simulink model "CCModel_73"  (R2024a)
settings: Solver=ode3  StartTime=0.0  StopTime=100  FixedStep=0.001  RelTol=1e-3  EnableMultiTasking=on
undefined symbols (not defined in the file or in its folder): DiscIntNeverNeededParam, Hecate_desVel1, Hecate_desVel2, Hecate_desVel3, Hecate_horShift, Hecate_period, Hecate_slope, Hecate_Transition1, Hecate_Transition2, Hecate_verShift, i, PME_qb, qb_map, RPM_qb, V
libraries: simulink x46
(part 2 of 11)

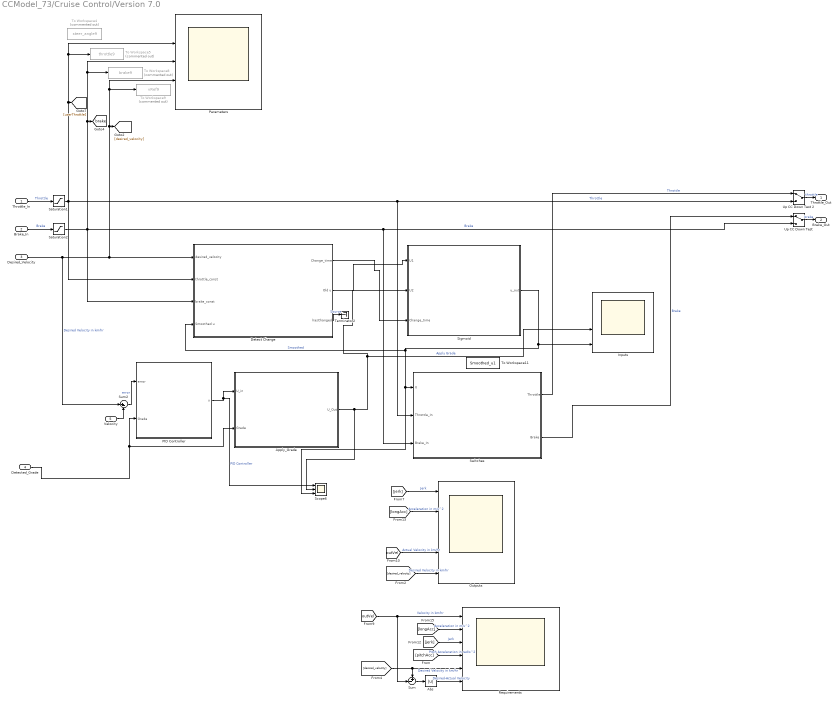
== system CCModel_73/Cruise Control/Version 7.0 ==
  Throttle_In : Inport
  Brake_In : Inport  Port=2
  Desired_Velocity : Inport  Port=3
  Detected_Grade : Inport  Port=4
  Velocity : Inport  Port=5
  Abs : Abs  SaturateOnIntegerOverflow=off
  Apply_Grade : Subsystem
  Detect Change : Subsystem
  Inputs : Scope  NumInputPorts=4
  Outputs : Scope  NumInputPorts=5
  PID Controller : Subsystem
  Parameters : Scope  NumInputPorts=5
  Requirements : Scope  NumInputPorts=6
  Saturation1 : Saturate  UpperLimit=100  LowerLimit=-100
  Saturation2 : Saturate  UpperLimit=100  LowerLimit=-100
  Scope6 : Scope  NumInputPorts=3
  Sigmoid : Subsystem
  Sum : Sum  Inputs=+-|
  Sum2 : Sum  Inputs=|+-
  Switches : Subsystem
  Terminator2 : Terminator
  To Workspace11 : ToWorkspace  VariableName=Smoothed_u1  SampleTime=-1
  To Workspace4 : ToWorkspace  Commented=on  VariableName=steer_angle9  SampleTime=-1
      settings: Save2DSignal=2-D array (concatenate along first dimension)
  To Workspace5 : ToWorkspace  Commented=on  VariableName=throttle9  SampleTime=-1
      settings: Save2DSignal=2-D array (concatenate along first dimension)
  To Workspace8 : ToWorkspace  Commented=on  VariableName=brake9  SampleTime=-1
      settings: Save2DSignal=2-D array (concatenate along first dimension)
  To Workspace9 : ToWorkspace  Commented=on  VariableName=vRef9  SampleTime=-1
      settings: Save2DSignal=2-D array (concatenate along first dimension)
  Up CC Down Test : ManualSwitch
  Up CC Down Test 2 : ManualSwitch
  Throttle_Out : Outport
  Brake_Out : Outport  Port=2
  tag scope: brake=global
  wires:
  Abs/1 -> Requirements/6  "Desired-Actual Velocity"
  Sum/1 -> Abs/1
  Switches/2(Brake) -> Up CC Down Test/1  "Brake"
  Saturation2/1 -> Switches/3(Brake_In), Up CC Down Test/2, Detect Change/3(brake_const), To Workspace8/1, Parameters/3, [brake]  "Brake"
  [jerk] -> Requirements/3  "Jerk"
  Detect Change/1(Change_time) -> Sigmoid/3(Change_time)
  Desired_Velocity/1 -> To Workspace9/1, Parameters/4, [desired_velocity], Detect Change/1(desired_velocity), Sum2/1  "Desired Velocity in km/hr"
  Sum2/1 -> PID Controller/1(error)  "error"
  Switches/1(Throttle) -> Up CC Down Test 2/1  "Throttle"
  PID Controller/1(u) -> Scope6/1, Apply_Grade/1(U_in)  "PID Controller"
  [outVel] -> Outputs/4  "Actual Velocity in km/hr"
  [longAcc] -> Outputs/2  "Acceleration in m/s^2"
  Throttle_In/1 -> Saturation1/1  "Throttle"
  [desired_velocity] -> Outputs/5  "Desired Velocity in km/hr"
  [longAcc] -> Requirements/2  "Acceleration in m/s^2"
  Up CC Down Test 2/1 -> Throttle_Out/1  "throttle"
  Velocity/1 -> Sum2/2
  [desired_velocity] -> Sum/1, Requirements/5  "Desired Velocity in km/hr"
  Detected_Grade/1 -> Apply_Grade/2(Grade), PID Controller/2(Grade)
  Brake_In/1 -> Saturation2/1  "Brake"
  Detect Change/3(hasChanged) -> Terminator2/1  "Source"
  Detect Change/2(Old u) -> Sigmoid/1(U1)
  Sigmoid/1(u_out) -> Detect Change/4(Smoothed u), Scope6/3, Switches/1(U), Inputs/4  "Smoothed"
  Apply_Grade/1(U_Out) -> Scope6/2, Inputs/3, Sigmoid/2(U2)  "Apply Grade"
  [pitchAcc] -> Requirements/4  "Pitch Acceleration in rad/s^2"
  [jerk] -> Outputs/1  "Jerk"
  Saturation1/1 -> Switches/2(Throttle_In), Up CC Down Test 2/2, Detect Change/2(throttle_const), [userThrottle], Parameters/2, To Workspace5/1  "Throttle"
  [outVel] -> Sum/2, Requirements/1  "Velocity in km/hr"
  Up CC Down Test/1 -> Brake_Out/1  "brake"

== system CCModel_73/Cruise Control/Version 7.1 ==
  Throttle_In : Inport
  Brake_In : Inport  Port=2
  Desired_Velocity : Inport  Port=3
  Detected_Grade : Inport  Port=4
  Velocity : Inport  Port=5
  Abs : Abs  SaturateOnIntegerOverflow=off
  Apply_Grade : Subsystem
  Detect Change : Subsystem
  Inputs : Scope  NumInputPorts=4
  Outputs : Scope  NumInputPorts=5
  PID Controller : Subsystem
  Parameters : Scope  NumInputPorts=5
  Requirements : Scope  NumInputPorts=6
  Saturation1 : Saturate  UpperLimit=100  LowerLimit=-100
  Saturation2 : Saturate  UpperLimit=100  LowerLimit=-100
  Scope6 : Scope  NumInputPorts=3
  Sigmoid : Subsystem
  Sum : Sum  Inputs=+-|
  Sum2 : Sum  Inputs=|+-
  Switches : Subsystem
  To Workspace4 : ToWorkspace  Commented=on  VariableName=steer_angle10  SampleTime=-1
      settings: Save2DSignal=2-D array (concatenate along first dimension)
  To Workspace5 : ToWorkspace  Commented=on  VariableName=throttle10  SampleTime=-1
      settings: Save2DSignal=2-D array (concatenate along first dimension)
  To Workspace8 : ToWorkspace  Commented=on  VariableName=brake10  SampleTime=-1
      settings: Save2DSignal=2-D array (concatenate along first dimension)
  To Workspace9 : ToWorkspace  Commented=on  VariableName=vRef10  SampleTime=-1
      settings: Save2DSignal=2-D array (concatenate along first dimension)
  Up CC Down Test : ManualSwitch
  Up CC Down Test 2 : ManualSwitch
  Throttle_Out : Outport
  Brake_Out : Outport  Port=2
  tag scope: ChangeTrigger=global, brake=global
  wires:
  PID Controller/1(u) -> Scope6/1, Apply_Grade/1(U_in)  "PID Controller"
  Detect Change/2(Old u) -> Sigmoid/1(U1)
  [longAcc] -> Outputs/2  "Acceleration in m/s^2"
  [desired_velocity] -> Outputs/5  "Desired Velocity in km/hr"
  Up CC Down Test 2/1 -> Throttle_Out/1  "throttle"
  Detect Change/1(Change_time) -> Sigmoid/3(Change_time)
  [outVel] -> Outputs/4  "Actual Velocity in km/hr"
  [desired_velocity] -> Sum/1, Requirements/5  "Desired Velocity in km/hr"
  [outVel] -> Sum/2, Requirements/1  "Velocity in km/hr"
  Velocity/1 -> Sum2/2
  [longAcc] -> Requirements/2  "Acceleration in m/s^2"
  Throttle_In/1 -> Saturation1/1  "Throttle"
  Abs/1 -> Requirements/6  "Desired-Actual Velocity"
  Switches/2(Brake) -> Up CC Down Test/1  "Brake"
  Sum/1 -> Abs/1
  Saturation2/1 -> Switches/3(Brake_In), Up CC Down Test/2, Detect Change/3(brake_const), To Workspace8/1, Parameters/3, [brake]  "Brake"
  Apply_Grade/1(U_Out) -> Scope6/2, Inputs/3, Sigmoid/2(U2)  "Apply Grade"
  [jerk] -> Requirements/3  "Jerk"
  [jerk] -> Outputs/1  "Jerk"
  Detect Change/3(hasChanged) -> [ChangeTrigger]  "Source"
  [pitchAcc] -> Requirements/4  "Pitch Acceleration in rad/s^2"
  Sum2/1 -> PID Controller/1(error)  "error"
  Switches/1(Throttle) -> Up CC Down Test 2/1  "Throttle"
  Brake_In/1 -> Saturation2/1  "Brake"
  Sigmoid/1(u_out) -> Detect Change/4(Smoothed u), Scope6/3, Switches/1(U), Inputs/4  "Smoothed"
  Desired_Velocity/1 -> To Workspace9/1, Parameters/4, [desired_velocity], Detect Change/1(desired_velocity), Sum2/1  "Desired Velocity in km/hr"
  Saturation1/1 -> [userThrottle], Parameters/2, To Workspace5/1, Switches/2(Throttle_In), Up CC Down Test 2/2, Detect Change/2(throttle_const)  "Throttle"
  Detected_Grade/1 -> Apply_Grade/2(Grade), PID Controller/2(Grade)
  Up CC Down Test/1 -> Brake_Out/1  "brake"

== system CCModel_73/Cruise Control/Version 7.2 ==
  Throttle_In : Inport
  Brake_In : Inport  Port=2
  Desired_Velocity : Inport  Port=3
  Detected_Grade : Inport  Port=4
  Velocity : Inport  Port=5
  Abs : Abs  SaturateOnIntegerOverflow=off
  Apply_Grade : Subsystem
  Detect Change : Subsystem
  Inputs : Scope  NumInputPorts=4
  PID Controller : Subsystem
  Parameters : Scope  NumInputPorts=5
  Requirements : Scope  NumInputPorts=6
  Saturation1 : Saturate  UpperLimit=100  LowerLimit=-100
  Saturation2 : Saturate  UpperLimit=100  LowerLimit=-100
  Scope6 : Scope  NumInputPorts=3
  Scope7 : Scope  NumInputPorts=5
  Sigmoid : Subsystem
  Sum : Sum  Inputs=+-|
  Sum2 : Sum  Inputs=|+-
  Switches : Subsystem
  To Workspace4 : ToWorkspace  Commented=on  VariableName=steer_angle11  SampleTime=-1
      settings: Save2DSignal=2-D array (concatenate along first dimension)
  To Workspace5 : ToWorkspace  Commented=on  VariableName=throttle11  SampleTime=-1
      settings: Save2DSignal=2-D array (concatenate along first dimension)
  To Workspace8 : ToWorkspace  Commented=on  VariableName=brake11  SampleTime=-1
      settings: Save2DSignal=2-D array (concatenate along first dimension)
  To Workspace9 : ToWorkspace  Commented=on  VariableName=vRef11  SampleTime=-1
      settings: Save2DSignal=2-D array (concatenate along first dimension)
  Up CC Down Test : ManualSwitch
  Up CC Down Test 2 : ManualSwitch
  Throttle_Out : Outport
  Brake_Out : Outport  Port=2
  tag scope: brake=global
  wires:
  [jerk] -> Scope7/1  "Jerk"
  [outVel] -> Scope7/4  "Actual Velocity in km/hr"
  [pitchAcc] -> Requirements/4  "Pitch Acceleration in rad/s^2"
  Up CC Down Test 2/1 -> Throttle_Out/1  "throttle"
  [longAcc] -> Requirements/2  "Acceleration in m/s^2"
  [outVel] -> Sum/2, Requirements/1  "Velocity in km/hr"
  Saturation1/1 -> Switches/2(Throttle_In), Up CC Down Test 2/2, Detect Change/2(throttle_const), [userThrottle], Parameters/2, To Workspace5/1  "Throttle"
  Velocity/1 -> Sum2/2
  [desired_velocity] -> Sum/1, Requirements/5  "Desired Velocity in km/hr"
  Detect Change/1(Change_time) -> Sigmoid/3(Change_time)
  Switches/2(Brake) -> Up CC Down Test/1  "Brake"
  Sum2/1 -> PID Controller/1(error)  "error"
  Desired_Velocity/1 -> To Workspace9/1, Parameters/4, [desired_velocity], Detect Change/1(desired_velocity), Sum2/1  "Desired Velocity in km/hr"
  Throttle_In/1 -> Saturation1/1  "Throttle"
  Switches/1(Throttle) -> Up CC Down Test 2/1  "Throttle"
  Saturation2/1 -> Switches/3(Brake_In), Up CC Down Test/2, Detect Change/3(brake_const), To Workspace8/1, Parameters/3, [brake]  "Brake"
  Detected_Grade/1 -> Apply_Grade/2(Grade), PID Controller/2(Grade)
  Sigmoid/1(u_out) -> Detect Change/4(Smoothed u), Scope6/3, Switches/1(U), Inputs/4  "Smoothed"
  Abs/1 -> Requirements/6  "Desired-Actual Velocity"
  [longAcc] -> Scope7/2  "Acceleration in m/s^2"
  Detect Change/3(hasChanged) -> Sigmoid/4(hasChanged)  "Source"
  Sum/1 -> Abs/1
  Brake_In/1 -> Saturation2/1  "Brake"
  PID Controller/1(u) -> Scope6/1, Apply_Grade/1(U_in)  "PID Controller"
  Detect Change/2(Old u) -> Sigmoid/1(U1)
  [desired_velocity] -> Scope7/5  "Desired Velocity in km/hr"
  Apply_Grade/1(U_Out) -> Scope6/2, Inputs/3, Sigmoid/2(U2)  "Apply Grade"
  [jerk] -> Requirements/3  "Jerk"
  Up CC Down Test/1 -> Brake_Out/1  "brake"

== system CCModel_73/Cruise Control/Version 7.3 ==
  Throttle_In : Inport
  Brake_In : Inport  Port=2
  Desired_Velocity : Inport  Port=3
  Detected_Grade : Inport  Port=4
  Velocity : Inport  Port=5
  Abs : Abs  SaturateOnIntegerOverflow=off
  Apply_Grade : Subsystem
  Detect Change : Subsystem
  Inputs : Scope  NumInputPorts=4
  Outputs : Scope  NumInputPorts=5
  PID Controller : Subsystem
  Parameters : Scope  NumInputPorts=5
  Requirements : Scope  NumInputPorts=6
  Saturation1 : Saturate  UpperLimit=100  LowerLimit=-100
  Saturation2 : Saturate  UpperLimit=100  LowerLimit=-100
  Scope6 : Scope  NumInputPorts=3
  Sigmoid : Subsystem
  Sum : Sum  Inputs=+-|
  Sum2 : Sum  Inputs=|+-
  Switches : Subsystem
  To Workspace18 : ToWorkspace  VariableName=Jerk  SampleTime=-1
      settings: Save2DSignal=2-D array (concatenate along first dimension)
  To Workspace4 : ToWorkspace  Commented=on  VariableName=steer_angle12  SampleTime=-1
      settings: Save2DSignal=2-D array (concatenate along first dimension)
  To Workspace5 : ToWorkspace  Commented=on  VariableName=throttle13  SampleTime=-1
      settings: Save2DSignal=2-D array (concatenate along first dimension)
  To Workspace8 : ToWorkspace  Commented=on  VariableName=brake12  SampleTime=-1
      settings: Save2DSignal=2-D array (concatenate along first dimension)
  To Workspace9 : ToWorkspace  Commented=on  VariableName=vRef12  SampleTime=-1
      settings: Save2DSignal=2-D array (concatenate along first dimension)
  Up CC Down Test : ManualSwitch
  Up CC Down Test 2 : ManualSwitch
  Throttle_Out : Outport
  Brake_Out : Outport  Port=2
  tag scope: ChangeTrigger=global, brake=global
  wires:
  Velocity/1 -> Sum2/2
  Sum2/1 -> Detect Change/5(error), PID Controller/1(Error)  "error"
  [jerk] -> Outputs/1  "Jerk"
  Switches/2(Brake) -> Up CC Down Test/1  "Brake"
  Switches/1(Throttle) -> Up CC Down Test 2/1  "Throttle"
  PID Controller/1(u) -> Scope6/1, Apply_Grade/1(U_in)  "PID Controller"
  Detect Change/3(hasChanged) -> PID Controller/2(Source)  "Source"
  [outVel] -> Outputs/4  "Actual Velocity in km/hr"
  [longAcc] -> Outputs/2  "Acceleration in m/s^2"
  [longAcc] -> Requirements/2  "Acceleration in m/s^2"
  Abs/1 -> Requirements/6  "Desired-Actual Velocity"
  [pitchAcc] -> Requirements/4  "Pitch Acceleration in rad/s^2"
  [jerk] -> To Workspace18/1, Requirements/3  "Jerk"
  [desired_velocity] -> Sum/1, Requirements/5  "Desired Velocity in km/hr"
  Saturation2/1 -> Switches/3(Brake_In), Up CC Down Test/2, Detect Change/3(brake_const), To Workspace8/1, Parameters/3, [brake]  "Brake"
  Detect Change/1(Change_time) -> Sigmoid/3(Change_time)
  [desired_velocity] -> Outputs/5  "Desired Velocity in km/hr"
  Detected_Grade/1 -> Apply_Grade/2(Grade)
  [outVel] -> Sum/2, Requirements/1  "Velocity in km/hr"
  Detect Change/2(Old u) -> Sigmoid/1(U1)  "Original"
  Brake_In/1 -> Saturation2/1  "Brake"
  Throttle_In/1 -> Saturation1/1  "Throttle"
  Sum/1 -> Abs/1
  Desired_Velocity/1 -> To Workspace9/1, Parameters/4, [desired_velocity], Detect Change/1(desired_velocity), PID Controller/3(Desired Velocity), Sum2/1  "Desired Velocity in km/hr"
  Up CC Down Test 2/1 -> Throttle_Out/1  "throttle"
  Sigmoid/1(u_out) -> Detect Change/4(Smoothed u), Scope6/3, Switches/1(U), Inputs/4  "Smoothed"
  Saturation1/1 -> Switches/2(Throttle_In), Up CC Down Test 2/2, Detect Change/2(throttle_const), [userThrottle], Parameters/2, To Workspace5/1  "Throttle"
  Apply_Grade/1(U_Out) -> Scope6/2, Inputs/3, Sigmoid/2(U2)  "Original"
  Up CC Down Test/1 -> Brake_Out/1  "brake"
  Detect Change/4(ChangeTrigger) -> [ChangeTrigger]

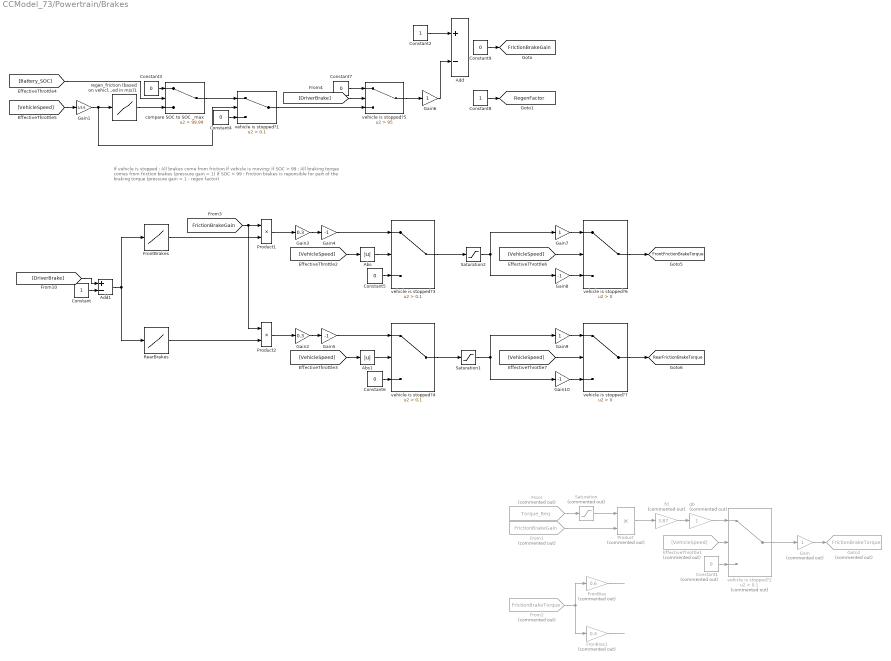
== system CCModel_73/Powertrain/Brakes ==
  note: If vehicle is stopped : All brakes come from friction
      | If vehicle is moving:
      | If SOC > 99 : All braking torque comes from friction brakes (pressure gain = 1)
      | If SOC < 99 : Friction brakes is reponsible for part of the braking torque (pressure gain = 1 - regen factor)
  Abs : Abs  SaturateOnIntegerOverflow=off
  Abs1 : Abs  SaturateOnIntegerOverflow=off
  Add : Sum  Inputs=+-
  Add1 : Sum  Inputs=+-
  Constant : Constant
  Constant1 : Constant  Commented=on  Value=0
  Constant2 : Constant
  Constant{3..7,9} (6 alike) : Constant  Value=0
  Constant8 : Constant
  EffectiveThrottle1 : From  Commented=on  GotoTag=VehicleSpeed  TagVisibility=global
      settings: CloseFcn=tagdialog Close
  From : From  Commented=on  GotoTag=Torque_Req  TagVisibility=global
  From1 : From  Commented=on  GotoTag=FrictionBrakeGain  TagVisibility=global
  From2 : From  Commented=on  GotoTag=FrictionBrakeTorque  TagVisibility=global
  FronBias : Gain  Commented=on  Gain=0.6
  FronBias1 : Gain  Commented=on  Gain=0.4
  FrontBrakes : Lookup_n-D  NumberOfTableDimensions=1  BreakpointsForDimension1=[0 10 20 30 40 50 60 70 80 90 100]  Table=[0 520 960 1390 1830 2260 2700 3140 3590 4030 4475]  InternalRulePriority=Speed  RndMeth=Simplest
  Gain : Gain  Commented=on
  Gain1 : Gain  Gain=1/3.6
  Gain{4..5,8,10} (4 alike) : Gain  Gain=-1
  Gain2 : Gain  Gain=0.3
  Gain3 : Gain  Gain=0.3
  Gain6 : Gain
  Gain7 : Gain
  Gain9 : Gain
  Goto2 : Goto  Commented=on  GotoTag=FrictionBrakeTorque  TagVisibility=global
  Product : Product  Commented=on
  Product1 : Product
  Product2 : Product
  RearBrakes : Lookup_n-D  NumberOfTableDimensions=1  BreakpointsForDimension1=[0 10 20 30 40 50 60 70 80 90 100]  Table=[0 170 250 340 420 500 580 664 740 825 905]  InternalRulePriority=Speed  RndMeth=Simplest
  Saturation : Saturate  Commented=on  UpperLimit=0  LowerLimit=-inf
  Saturation1 : Saturate  UpperLimit=0  LowerLimit=-inf
  Saturation2 : Saturate  UpperLimit=0  LowerLimit=-inf
  compare SOC to SOC _max : Switch  Criteria=u2 > Threshold  Threshold=99.99  SaturateOnIntegerOverflow=off  InputSameDT=off
  fd : Gain  Commented=on  Gain=3.87
  gb : Gain  Commented=on
  regen_friction (based on vehicle speed in m/s)1 : Lookup_n-D  NumberOfTableDimensions=1  BreakpointsForDimension1=[0,2.76,5.55,8.31,11.07,13.83,16.68,27.76,300]  Table="[0\t0.25  0.25\t0.25\t  0.50\t0.95\t0.95\t0.95   0.95]"  InternalRulePriority=Speed  RndMeth=Simplest
  vehicle is stopped?1 : Switch  Criteria=u2 > Threshold  Threshold=0.1  SaturateOnIntegerOverflow=off  InputSameDT=off
  vehicle is stopped?2 : Switch  Commented=on  Criteria=u2 > Threshold  Threshold=0.1  SaturateOnIntegerOverflow=off  InputSameDT=off
  vehicle is stopped?3 : Switch  Criteria=u2 > Threshold  Threshold=0.1  SaturateOnIntegerOverflow=off  InputSameDT=off
  vehicle is stopped?4 : Switch  Criteria=u2 > Threshold  Threshold=0.1  SaturateOnIntegerOverflow=off  InputSameDT=off
  vehicle is stopped?5 : Switch  Criteria=u2 > Threshold  Threshold=95  SaturateOnIntegerOverflow=off  InputSameDT=off
  vehicle is stopped?6 : Switch  Criteria=u2 > Threshold  SaturateOnIntegerOverflow=off  InputSameDT=off
  vehicle is stopped?7 : Switch  Criteria=u2 > Threshold  SaturateOnIntegerOverflow=off  InputSameDT=off
  tag scope: FrictionBrakeGain=global, FrontFrictionBrakeTorque=global, RearFrictionBrakeTorque=global, RegenFactor=global
  wires:
  [VehicleSpeed] -> Gain1/1
  Gain1/1 -> vehicle is stopped?1/2, regen_friction (based on vehicle speed in m/s)1/1
  Constant2/1 -> Add/1
  Constant3/1 -> compare SOC to SOC _max/1
  compare SOC to SOC _max/1 -> vehicle is stopped?1/1
  [Battery_SOC] -> compare SOC to SOC _max/2
  Constant4/1 -> vehicle is stopped?1/3
  EffectiveThrottle1/1 -> vehicle is stopped?2/2
  From1/1 -> Product/2
  fd/1 -> gb/1
  FronBias/1 -> ?
  FronBias1/1 -> ?
  From2/1 -> FronBias/1, FronBias1/1
  Saturation/1 -> Product/1
  gb/1 -> vehicle is stopped?2/1
  Constant1/1 -> vehicle is stopped?2/3
  vehicle is stopped?2/1 -> Gain/1
  From/1 -> Saturation/1
  Product/1 -> fd/1
  Gain/1 -> Goto2/1
  regen_friction (based on vehicle speed in m/s)1/1 -> compare SOC to SOC _max/3
  Add1/1 -> RearBrakes/1, FrontBrakes/1
  FrontBrakes/1 -> Product1/2
  RearBrakes/1 -> Product2/2
  [FrictionBrakeGain] -> Product2/1, Product1/1
  Product1/1 -> Gain3/1
  Product2/1 -> Gain2/1
  Gain2/1 -> Gain5/1
  Gain3/1 -> Gain4/1
  Constant/1 -> Add1/2
  [DriverBrake] -> Add1/1
  Gain6/1 -> Add/2
  [DriverBrake] -> vehicle is stopped?5/2
  vehicle is stopped?1/1 -> vehicle is stopped?5/3
  Constant7/1 -> vehicle is stopped?5/1
  vehicle is stopped?5/1 -> Gain6/1
  Abs1/1 -> vehicle is stopped?4/2
  Constant5/1 -> vehicle is stopped?3/3
  vehicle is stopped?7/1 -> [RearFrictionBrakeTorque]
  [VehicleSpeed] -> vehicle is stopped?7/2
  Gain10/1 -> vehicle is stopped?7/3
  Saturation1/1 -> Gain9/1, Gain10/1
  Saturation2/1 -> Gain8/1, Gain7/1
  Gain8/1 -> vehicle is stopped?6/3
  [VehicleSpeed] -> vehicle is stopped?6/2
  vehicle is stopped?4/1 -> Saturation1/1
  Gain9/1 -> vehicle is stopped?7/1
  Gain4/1 -> vehicle is stopped?3/1
  vehicle is stopped?3/1 -> Saturation2/1
  Gain7/1 -> vehicle is stopped?6/1
  Constant6/1 -> vehicle is stopped?4/3
  Abs/1 -> vehicle is stopped?3/2
  Gain5/1 -> vehicle is stopped?4/1
  vehicle is stopped?6/1 -> [FrontFrictionBrakeTorque]
  [VehicleSpeed] -> Abs/1
  [VehicleSpeed] -> Abs1/1
  Constant8/1 -> [RegenFactor]
  Constant9/1 -> [FrictionBrakeGain]

== system CCModel_73/Powertrain/Central Differential ==
  0 : Constant
  "1 " : Constant  Value=0
  Add : Sum  Inputs=+++
  Central Differential Active : Constant  Value=CentralDifferentialActive
  Constant : Constant
  Front Bias : Constant  Value=FrontBias
  Gain : Gain  Gain=0.5
  Gain1 : Gain  Gain=0.5
  Gain2 : Gain  Gain=0.5
  Product : Product
  Product1 : Product
  Sum : Sum  Inputs=-+|
  Sum1 : Sum
  Sum2 : Sum
  Sum3 : Sum
  Switch : Switch  Criteria=u2 > Threshold  SaturateOnIntegerOverflow=off  InputSameDT=off
  prod{,1..4} (5 alike) : Product
  tag scope: DiffFrontInputTorque=global, DiffRearInputTorque=global, GearboxOutputAlpha=global, GearboxOutputAngle=global, GearboxOutputOmega=global, InternalCentralDiffActivity=global
  wires:
  Front Bias/1 -> Sum/1, Product/2
  Constant/1 -> Sum/2
  Sum/1 -> Product1/2
  Add/1 -> Product1/1, Product/1
  Sum1/1 -> Gain/1
  [DiffRearInputOmega] -> Sum1/2
  [DiffFrontInputOmega] -> Sum1/1
  Sum2/1 -> Gain1/1
  [DiffRearInputAlpha] -> Sum2/2
  [DiffFrontInputAlpha] -> Sum2/1
  Sum3/1 -> Gain2/1
  [DiffRearInputAngle] -> Sum3/2
  [DiffFrontInputAngle] -> Sum3/1
  Central Differential Active/1 -> Switch/2, prod4/1, prod3/1, prod2/1, prod1/1, prod/1
  prod1/1 -> [DiffRearInputTorque]
  prod2/1 -> [GearboxOutputOmega]
  prod3/1 -> [GearboxOutputAlpha]
  prod4/1 -> [GearboxOutputAngle]
  Product/1 -> prod/2
  Product1/1 -> prod1/2
  Gain/1 -> prod2/2
  Gain1/1 -> prod3/2
  Gain2/1 -> prod4/2
  Switch/1 -> [InternalCentralDiffActivity]
  "1 "/1 -> Switch/1
  0/1 -> Switch/3
  [EM3Torque] -> Add/2
  [EVTorque] -> Add/3
  [DiffCenterInputshaftTorque] -> Add/1
  prod/1 -> [DiffFrontInputTorque]

== system CCModel_73/Powertrain/Clutch ==
  0 : Constant
  "1 " : Constant  Value=0
  Add : Sum  Inputs=+++
  Clutch Active : Constant  Value=ClutchActive
  Clutch Closed : Constant
  Clutch Omega : Product
  Constant1 : Constant  Value=0
  Gearbox Omega : Product
  GearboxAlpha : From  Commented=on  GotoTag=GearboxAlpha  TagVisibility=global
      settings: CloseFcn=tagdialog Close
  GearboxAngle : From  Commented=on  GotoTag=GearboxAngle  TagVisibility=global
      settings: CloseFcn=tagdialog Close
  Inertia to Accel : Gain  Gain=1/0.1
  Saturation : Saturate  UpperLimit=0  LowerLimit=-1000000
  Scope : Scope  Commented=on  NumInputPorts=2
  Sum : Sum
  Sum1 : Sum  Inputs=|++
  Sum2 : Sum  Inputs=+-  SaturateOnIntegerOverflow=on
  Switch : Switch  Criteria=u2 > Threshold  SaturateOnIntegerOverflow=off  InputSameDT=off
  Torque : Product
  "Vicrt Integration Time Step " : Gain  Gain=0.001
  prod : Product
  prod1 : Product
  tag scope: ClutchInputAlpha=global, ClutchInputAngle=global, ClutchInputOmega=global, GearboxInputTorque=global, InternalClutchActivity=global
  wires:
  [ClutchDemand] -> Sum2/2, Clutch Omega/1
  Inertia to Accel/1 -> "Vicrt Integration Time Step "/1
  Clutch Closed/1 -> Sum2/1
  Sum2/1 -> Gearbox Omega/1, Torque/2
  Gearbox Omega/1 -> Sum/1
  [GearboxOmega] -> Gearbox Omega/2
  [EngineOmega] -> Clutch Omega/2
  Clutch Omega/1 -> Sum/2
  Add/1 -> Torque/1, Inertia to Accel/1
  Sum/1 -> Sum1/1
  "Vicrt Integration Time Step "/1 -> Saturation/1
  Saturation/1 -> Sum1/2
  GearboxAlpha/1 -> Scope/1
  GearboxAngle/1 -> Scope/2
  Constant1/1 -> [ClutchInputAlpha], [ClutchInputAngle]
  prod/1 -> [GearboxInputTorque]
  prod1/1 -> [ClutchInputOmega]
  Sum1/1 -> prod1/2
  Torque/1 -> prod/2
  Clutch Active/1 -> prod1/1, prod/1, Switch/2
  "1 "/1 -> Switch/1
  0/1 -> Switch/3
  Switch/1 -> [InternalClutchActivity]
  [ClutchInputplateTorque] -> Add/1
  [EM1Torque] -> Add/2
  [EM0Torque] -> Add/3

== system CCModel_73/Powertrain/EM0 ==
  note: If Torque is positive: Motor does its best
      | If torque is negative: Case 01: SOC > 99: No Regen (Tmot = 0)
      | Case 02: SOC < 99: Regen
      | If Vehicle is stopped: No Regen Brakes
  0 : Constant
  "1 " : Constant  Value=0
  Constant1 : Constant  Value=0
  EM0 Active : Constant  Value=EM0Active
  EM0ConectionRatio : Constant  Value=EM0_Ratio
  Memory1 : Memory  InheritSampleTime=on
  Negative Motor Torque Table : Lookup_n-D  NumberOfTableDimensions=1  BreakpointsForDimension1=|  Table=|  InternalRulePriority=Speed  RndMeth=Simplest
      BreakpointsForDimension1=|
      | [1
      | 300
      | 700
      | 1000
      | 1300
      | 1600
      | 1900
      | 2200
      | 2500
      | 2800
      | 3100
      | 3400
      | 3700
      | 4000
      | 4300
      | 4600
      | 4900
      | 5200
      | 5500
      | 5800
      | 6100
      | 6400
      | 6700
      | 7000
      | 7400
      | 7800
      | 8200
      | 8600
      | 8810]
      Table=|
      | [-360
      | -360
      | -360
      | -360
      | -360
      | -357.728404316261
      | -357.682405078656
      | -356.960983702214
      | -356.300227986961
      | -355.518140949330
      | -355.472141711725
      | -351.285699987009
      | -343.284814075766
      | -334.455149023278
      | -326.397812480700
      | -307.963362459085
      | -289.161940741908
      | -276.934802218937
      | -265.691686602383
      | -254.400604378871
      | -242.676261199004
      | -229.462130210989
      | -218.075437684875
      | -207.776256300937
      | -192.222891861329
      | -178.005775209291
      | -168.578005975641
      | -157.192637101830
      | -152.195121951219]
  Positive Motor Torque Table : Lookup_n-D  NumberOfTableDimensions=1  BreakpointsForDimension1=|  Table=|  InternalRulePriority=Speed  RndMeth=Simplest
      BreakpointsForDimension1=|
      | [1
      | 300
      | 700
      | 1000
      | 1300
      | 1600
      | 1900
      | 2200
      | 2500
      | 2800
      | 3100
      | 3400
      | 3700
      | 4000
      | 4300
      | 4600
      | 4900
      | 5200
      | 5500
      | 5800
      | 6100
      | 6400
      | 6700
      | 7000
      | 7400
      | 7800
      | 8200
      | 8600
      | 8810]
      Table=|
      | [360
      | 360
      | 360
      | 360
      | 360
      | 357.728404316261
      | 357.682405078656
      | 356.960983702214
      | 356.300227986961
      | 355.518140949330
      | 355.472141711725
      | 351.285699987009
      | 343.284814075766
      | 334.455149023278
      | 326.397812480700
      | 307.963362459085
      | 289.161940741908
      | 276.934802218937
      | 265.691686602383
      | 254.400604378871
      | 242.676261199004
      | 229.462130210989
      | 218.075437684875
      | 207.776256300937
      | 192.222891861329
      | 178.005775209291
      | 168.578005975641
      | 157.192637101830
      | 152.195121951219]
  Product : Product
  Saturation Dynamic1 : simulink/Discontinuities/Saturation Dynamic  OutMin=[-360]  OutMax=[360]  OutDataTypeStr=Inherit: Same as second input  OutDataType=fixdt(1, 16)  OutScaling=2^-10  DoSatur=off
  Switch : Switch  Criteria=u2 > Threshold  SaturateOnIntegerOverflow=off  InputSameDT=off
  Switch3 : Switch  SaturateOnIntegerOverflow=off  InputSameDT=off
  compare SOC to SOC _max : Switch  Criteria=u2 > Threshold  Threshold=99  SaturateOnIntegerOverflow=off  InputSameDT=off
  efficiency : Subsystem
  prod : Product
  prod1 : Product
  rad_sec_to_rpm : Gain  Gain=60/2/pi
  tag scope: EM0BeltRatio=global, EM0Torque=global, EM0_ElectricPower_W=global, InternalEM0Activity=global
  wires:
  Switch/1 -> [InternalEM0Activity]
  "1 "/1 -> Switch/1
  0/1 -> Switch/3
  [EM0TorqueCmd] -> Saturation Dynamic1/2
  efficiency/1(Electrical power [W]) -> prod1/1
  Constant1/1 -> compare SOC to SOC _max/1
  Memory1/1 -> Negative Motor Torque Table/1, Positive Motor Torque Table/1
  compare SOC to SOC _max/1 -> Switch3/3
  [EM0Omega] -> rad_sec_to_rpm/1
  Saturation Dynamic1/1 -> Switch3/2, Switch3/1, compare SOC to SOC _max/3
  rad_sec_to_rpm/1 -> efficiency/1(Motor speed [rpm]), Memory1/1
  Negative Motor Torque Table/1 -> Saturation Dynamic1/3
  [SOC] -> compare SOC to SOC _max/2
  Switch3/1 -> prod/1
  prod/1 -> Product/1, efficiency/2("Torque [Nm] ")
  Positive Motor Torque Table/1 -> Saturation Dynamic1/1
  prod1/1 -> [EM0_ElectricPower_W]
  EM0 Active/1 -> Switch/2, prod1/2, prod/2
  Product/1 -> [EM0Torque]
  EM0ConectionRatio/1 -> [EM0BeltRatio], Product/2

== system CCModel_73/Powertrain/EM1 ==
  note: If Torque is positive: Motor does its best
      | If torque is negative: Case 01: SOC > 99: No Regen (Tmot = 0)
      | Case 02: SOC < 99: Regen
      | If Vehicle is stopped: No Regen Brakes
  0 : Constant
  "1 " : Constant  Value=0
  Constant1 : Constant  Value=0
  EM1 Active : Constant  Value=EM1Active
  EM1ConectionRatio : Constant  Value=EM1_Ratio
  Memory1 : Memory  InheritSampleTime=on
  Negative Motor Torque Table : Lookup_n-D  NumberOfTableDimensions=1  BreakpointsForDimension1=|  Table=|  InternalRulePriority=Speed  RndMeth=Simplest
      BreakpointsForDimension1=|
      | [1
      | 300
      | 700
      | 1000
      | 1300
      | 1600
      | 1900
      | 2200
      | 2500
      | 2800
      | 3100
      | 3400
      | 3700
      | 4000
      | 4300
      | 4600
      | 4900
      | 5200
      | 5500
      | 5800
      | 6100
      | 6400
      | 6700
      | 7000
      | 7400
      | 7800
      | 8200
      | 8600
      | 8810]
      Table=|
      | [-360
      | -360
      | -360
      | -360
      | -360
      | -357.728404316261
      | -357.682405078656
      | -356.960983702214
      | -356.300227986961
      | -355.518140949330
      | -355.472141711725
      | -351.285699987009
      | -343.284814075766
      | -334.455149023278
      | -326.397812480700
      | -307.963362459085
      | -289.161940741908
      | -276.934802218937
      | -265.691686602383
      | -254.400604378871
      | -242.676261199004
      | -229.462130210989
      | -218.075437684875
      | -207.776256300937
      | -192.222891861329
      | -178.005775209291
      | -168.578005975641
      | -157.192637101830
      | -152.195121951219]
  Positive Motor Torque Table : Lookup_n-D  NumberOfTableDimensions=1  BreakpointsForDimension1=|  Table=|  InternalRulePriority=Speed  RndMeth=Simplest
      BreakpointsForDimension1=|
      | [1
      | 300
      | 700
      | 1000
      | 1300
      | 1600
      | 1900
      | 2200
      | 2500
      | 2800
      | 3100
      | 3400
      | 3700
      | 4000
      | 4300
      | 4600
      | 4900
      | 5200
      | 5500
      | 5800
      | 6100
      | 6400
      | 6700
      | 7000
      | 7400
      | 7800
      | 8200
      | 8600
      | 8810]
      Table=|
      | [360
      | 360
      | 360
      | 360
      | 360
      | 357.728404316261
      | 357.682405078656
      | 356.960983702214
      | 356.300227986961
      | 355.518140949330
      | 355.472141711725
      | 351.285699987009
      | 343.284814075766
      | 334.455149023278
      | 326.397812480700
      | 307.963362459085
      | 289.161940741908
      | 276.934802218937
      | 265.691686602383
      | 254.400604378871
      | 242.676261199004
      | 229.462130210989
      | 218.075437684875
      | 207.776256300937
      | 192.222891861329
      | 178.005775209291
      | 168.578005975641
      | 157.192637101830
      | 152.195121951219]
  Product : Product
  Saturation Dynamic1 : simulink/Discontinuities/Saturation Dynamic  OutMin=[-360]  OutMax=[360]  OutDataTypeStr=Inherit: Same as second input  OutDataType=fixdt(1, 16)  OutScaling=2^-10  DoSatur=off
  Switch : Switch  Criteria=u2 > Threshold  SaturateOnIntegerOverflow=off  InputSameDT=off
  Switch3 : Switch  SaturateOnIntegerOverflow=off  InputSameDT=off
  compare SOC to SOC _max : Switch  Criteria=u2 > Threshold  Threshold=99  SaturateOnIntegerOverflow=off  InputSameDT=off
  efficiency : Subsystem
  prod : Product
  prod1 : Product
  rad_sec_to_rpm : Gain  Gain=60/2/pi
  tag scope: EM1BeltRatio=global, EM1Torque=global, EM1_ElectricPower_W=global, InternalEM1Activity=global
  wires:
  Switch/1 -> [InternalEM1Activity]
  "1 "/1 -> Switch/1
  0/1 -> Switch/3
  Product/1 -> [EM1Torque]
  prod1/1 -> [EM1_ElectricPower_W]
  [SOC] -> compare SOC to SOC _max/2
  rad_sec_to_rpm/1 -> efficiency/1(Motor speed [rpm]), Memory1/1
  Switch3/1 -> prod/1
  Negative Motor Torque Table/1 -> Saturation Dynamic1/3
  Saturation Dynamic1/1 -> Switch3/2, Switch3/1, compare SOC to SOC _max/3
  Positive Motor Torque Table/1 -> Saturation Dynamic1/1
  [EM1Omega] -> rad_sec_to_rpm/1
  Memory1/1 -> Negative Motor Torque Table/1, Positive Motor Torque Table/1
  Constant1/1 -> compare SOC to SOC _max/1
  [EM1TorqueCmd] -> Saturation Dynamic1/2
  EM1 Active/1 -> prod1/2, prod/2, Switch/2
  efficiency/1(Electrical power [W]) -> prod1/1
  EM1ConectionRatio/1 -> [EM1BeltRatio], Product/2
  prod/1 -> efficiency/2("Torque [Nm] "), Product/1
  compare SOC to SOC _max/1 -> Switch3/3

== system CCModel_73/Powertrain/EM2 ==
  note: If Torque is positive: Motor does its best
      | If torque is negative: Case 01: SOC > 99: No Regen (Tmot = 0)
      | Case 02: SOC < 99: Regen
      | If Vehicle is stopped: No Regen Brakes
  0 : Constant
  "1 " : Constant  Value=0
  EM2 Active : Constant  Value=EM2Active
  Memory1 : Memory  InheritSampleTime=on
  Negative Motor Torque Table : Lookup_n-D  NumberOfTableDimensions=1  BreakpointsForDimension1=|  Table=|  InternalRulePriority=Speed  RndMeth=Simplest
      BreakpointsForDimension1=|
      | [1
      | 300
      | 700
      | 1000
      | 1300
      | 1600
      | 1900
      | 2200
      | 2500
      | 2800
      | 3100
      | 3400
      | 3700
      | 4000
      | 4300
      | 4600
      | 4900
      | 5200
      | 5500
      | 5800
      | 6100
      | 6400
      | 6700
      | 7000
      | 7400
      | 7800
      | 8200
      | 8600
      | 8810]
      Table=|
      | [-360
      | -360
      | -360
      | -360
      | -360
      | -357.728404316261
      | -357.682405078656
      | -356.960983702214
      | -356.300227986961
      | -355.518140949330
      | -355.472141711725
      | -351.285699987009
      | -343.284814075766
      | -334.455149023278
      | -326.397812480700
      | -307.963362459085
      | -289.161940741908
      | -276.934802218937
      | -265.691686602383
      | -254.400604378871
      | -242.676261199004
      | -229.462130210989
      | -218.075437684875
      | -207.776256300937
      | -192.222891861329
      | -178.005775209291
      | -168.578005975641
      | -157.192637101830
      | -152.195121951219]
  Positive Motor Torque Table : Lookup_n-D  NumberOfTableDimensions=1  BreakpointsForDimension1=|  Table=|  InternalRulePriority=Speed  RndMeth=Simplest
      BreakpointsForDimension1=|
      | [1
      | 300
      | 700
      | 1000
      | 1300
      | 1600
      | 1900
      | 2200
      | 2500
      | 2800
      | 3100
      | 3400
      | 3700
      | 4000
      | 4300
      | 4600
      | 4900
      | 5200
      | 5500
      | 5800
      | 6100
      | 6400
      | 6700
      | 7000
      | 7400
      | 7800
      | 8200
      | 8600
      | 8810]
      Table=|
      | [360
      | 360
      | 360
      | 360
      | 360
      | 357.728404316261
      | 357.682405078656
      | 356.960983702214
      | 356.300227986961
      | 355.518140949330
      | 355.472141711725
      | 351.285699987009
      | 343.284814075766
      | 334.455149023278
      | 326.397812480700
      | 307.963362459085
      | 289.161940741908
      | 276.934802218937
      | 265.691686602383
      | 254.400604378871
      | 242.676261199004
      | 229.462130210989
      | 218.075437684875
      | 207.776256300937
      | 192.222891861329
      | 178.005775209291
      | 168.578005975641
      | 157.192637101830
      | 152.195121951219]
  Saturation Dynamic1 : simulink/Discontinuities/Saturation Dynamic  OutMin=[-360]  OutMax=[360]  OutDataTypeStr=Inherit: Same as second input  OutDataType=fixdt(1, 16)  OutScaling=2^-10  DoSatur=off
  Switch : Switch  Criteria=u2 > Threshold  SaturateOnIntegerOverflow=off  InputSameDT=off
  Switch3 : Switch  SaturateOnIntegerOverflow=off  InputSameDT=off
  efficiency : Subsystem
  prod : Product
  prod1 : Product
  prod2 : Product
  rad_sec_to_rpm : Gain  Gain=60/2/pi
  tag scope: EM2Torque=global, EM2_ElectricPower_W=global, InternalEM2Activity=global
  wires:
  EM2 Active/1 -> prod1/2, prod/2, Switch/2
  Switch/1 -> [InternalEM2Activity]
  "1 "/1 -> Switch/1
  0/1 -> Switch/3
  prod/1 -> efficiency/2("Torque [Nm] "), [EM2Torque]
  Switch3/1 -> prod/1
  Negative Motor Torque Table/1 -> Saturation Dynamic1/3
  Positive Motor Torque Table/1 -> Saturation Dynamic1/1
  Saturation Dynamic1/1 -> prod2/1, Switch3/2, Switch3/1
  [EM2Omega] -> rad_sec_to_rpm/1
  Memory1/1 -> Negative Motor Torque Table/1, Positive Motor Torque Table/1
  prod2/1 -> Switch3/3
  [EM2TorqueCmd] -> Saturation Dynamic1/2
  rad_sec_to_rpm/1 -> efficiency/1(Motor speed [rpm]), Memory1/1
  efficiency/1(Electrical power [W]) -> prod1/1
  prod1/1 -> [EM2_ElectricPower_W]
  [RegenFactor] -> prod2/2

== system CCModel_73/Powertrain/EM3 ==
  note: If Torque is positive: Motor does its best
      | If torque is negative: Case 01: SOC > 99: No Regen (Tmot = 0)
      | Case 02: SOC < 99: Regen
      | If Vehicle is stopped: No Regen Brakes
  0 : Constant
  "1 " : Constant  Value=0
  Belt_Ratio : Gain
  EM3 Active : Constant  Value=EM3Active
  Memory1 : Memory  InheritSampleTime=on
  Negative Motor Torque Table : Lookup_n-D  NumberOfTableDimensions=1  BreakpointsForDimension1=|  Table=|  InternalRulePriority=Speed  RndMeth=Simplest
      BreakpointsForDimension1=|
      | [1
      | 300
      | 700
      | 1000
      | 1300
      | 1600
      | 1900
      | 2200
      | 2500
      | 2800
      | 3100
      | 3400
      | 3700
      | 4000
      | 4300
      | 4600
      | 4900
      | 5200
      | 5500
      | 5800
      | 6100
      | 6400
      | 6700
      | 7000
      | 7400
      | 7800
      | 8200
      | 8600
      | 8810]
      Table=|
      | [-360
      | -360
      | -360
      | -360
      | -360
      | -357.728404316261
      | -357.682405078656
      | -356.960983702214
      | -356.300227986961
      | -355.518140949330
      | -355.472141711725
      | -351.285699987009
      | -343.284814075766
      | -334.455149023278
      | -326.397812480700
      | -307.963362459085
      | -289.161940741908
      | -276.934802218937
      | -265.691686602383
      | -254.400604378871
      | -242.676261199004
      | -229.462130210989
      | -218.075437684875
      | -207.776256300937
      | -192.222891861329
      | -178.005775209291
      | -168.578005975641
      | -157.192637101830
      | -152.195121951219]
  Positive Motor Torque Table : Lookup_n-D  NumberOfTableDimensions=1  BreakpointsForDimension1=|  Table=|  InternalRulePriority=Speed  RndMeth=Simplest
      BreakpointsForDimension1=|
      | [1
      | 300
      | 700
      | 1000
      | 1300
      | 1600
      | 1900
      | 2200
      | 2500
      | 2800
      | 3100
      | 3400
      | 3700
      | 4000
      | 4300
      | 4600
      | 4900
      | 5200
      | 5500
      | 5800
      | 6100
      | 6400
      | 6700
      | 7000
      | 7400
      | 7800
      | 8200
      | 8600
      | 8810]
      Table=|
      | [360
      | 360
      | 360
      | 360
      | 360
      | 357.728404316261
      | 357.682405078656
      | 356.960983702214
      | 356.300227986961
      | 355.518140949330
      | 355.472141711725
      | 351.285699987009
      | 343.284814075766
      | 334.455149023278
      | 326.397812480700
      | 307.963362459085
      | 289.161940741908
      | 276.934802218937
      | 265.691686602383
      | 254.400604378871
      | 242.676261199004
      | 229.462130210989
      | 218.075437684875
      | 207.776256300937
      | 192.222891861329
      | 178.005775209291
      | 168.578005975641
      | 157.192637101830
      | 152.195121951219]
  Saturation Dynamic1 : simulink/Discontinuities/Saturation Dynamic  OutMin=[-360]  OutMax=[360]  OutDataTypeStr=Inherit: Same as second input  OutDataType=fixdt(1, 16)  OutScaling=2^-10  DoSatur=off
  Switch : Switch  Criteria=u2 > Threshold  SaturateOnIntegerOverflow=off  InputSameDT=off
  Switch3 : Switch  SaturateOnIntegerOverflow=off  InputSameDT=off
  efficiency : Subsystem
  prod : Product
  prod1 : Product
  prod2 : Product
  rad_sec_to_rpm : Gain  Gain=60/2/pi
  tag scope: EM3Torque=global, EM3_ElectricPower_W=global, InternalEM3Activity=global
  wires:
  Switch/1 -> [InternalEM3Activity]
  "1 "/1 -> Switch/1
  0/1 -> Switch/3
  EM3 Active/1 -> prod1/2, prod/2, Switch/2
  Memory1/1 -> Negative Motor Torque Table/1, Positive Motor Torque Table/1
  [EM3TorqueCmd] -> Saturation Dynamic1/2
  efficiency/1(Electrical power [W]) -> prod1/1
  Saturation Dynamic1/1 -> prod2/1, Switch3/2, Switch3/1
  [EM3Omega] -> rad_sec_to_rpm/1
  prod2/1 -> Switch3/3
  Positive Motor Torque Table/1 -> Saturation Dynamic1/1
  Switch3/1 -> prod/1
  Negative Motor Torque Table/1 -> Saturation Dynamic1/3
  rad_sec_to_rpm/1 -> efficiency/1(Motor speed [rpm]), Memory1/1
  prod1/1 -> [EM3_ElectricPower_W]
  prod/1 -> efficiency/2("Torque [Nm] "), Belt_Ratio/1
  Belt_Ratio/1 -> [EM3Torque]
  [RegenFactor] -> prod2/2

== system CCModel_73/Powertrain/EM4Front ==
  note: If Torque is positive: Motor does its best
      | If torque is negative: Case 01: SOC > 99: No Regen (Tmot = 0)
      | Case 02: SOC < 99: Regen
      | If Vehicle is stopped: No Regen Brakes
  0 : Constant
  "1 " : Constant  Value=0
  Belt_Ratio : Gain
  EM4 Front Active : Constant  Value=EM4FrontActive
  Memory1 : Memory  InheritSampleTime=on
  Negative Motor Torque Table : Lookup_n-D  NumberOfTableDimensions=1  BreakpointsForDimension1=|  Table=|  InternalRulePriority=Speed  RndMeth=Simplest
      BreakpointsForDimension1=|
      | [1
      | 300
      | 700
      | 1000
      | 1300
      | 1600
      | 1900
      | 2200
      | 2500
      | 2800
      | 3100
      | 3400
      | 3700
      | 4000
      | 4300
      | 4600
      | 4900
      | 5200
      | 5500
      | 5800
      | 6100
      | 6400
      | 6700
      | 7000
      | 7400
      | 7800
      | 8200
      | 8600
      | 8810]
      Table=|
      | [-360
      | -360
      | -360
      | -360
      | -360
      | -357.728404316261
      | -357.682405078656
      | -356.960983702214
      | -356.300227986961
      | -355.518140949330
      | -355.472141711725
      | -351.285699987009
      | -343.284814075766
      | -334.455149023278
      | -326.397812480700
      | -307.963362459085
      | -289.161940741908
      | -276.934802218937
      | -265.691686602383
      | -254.400604378871
      | -242.676261199004
      | -229.462130210989
      | -218.075437684875
      | -207.776256300937
      | -192.222891861329
      | -178.005775209291
      | -168.578005975641
      | -157.192637101830
      | -152.195121951219]
  Positive Motor Torque Table : Lookup_n-D  NumberOfTableDimensions=1  BreakpointsForDimension1=|  Table=|  InternalRulePriority=Speed  RndMeth=Simplest
      BreakpointsForDimension1=|
      | [1
      | 300
      | 700
      | 1000
      | 1300
      | 1600
      | 1900
      | 2200
      | 2500
      | 2800
      | 3100
      | 3400
      | 3700
      | 4000
      | 4300
      | 4600
      | 4900
      | 5200
      | 5500
      | 5800
      | 6100
      | 6400
      | 6700
      | 7000
      | 7400
      | 7800
      | 8200
      | 8600
      | 8810]
      Table=|
      | [360
      | 360
      | 360
      | 360
      | 360
      | 357.728404316261
      | 357.682405078656
      | 356.960983702214
      | 356.300227986961
      | 355.518140949330
      | 355.472141711725
      | 351.285699987009
      | 343.284814075766
      | 334.455149023278
      | 326.397812480700
      | 307.963362459085
      | 289.161940741908
      | 276.934802218937
      | 265.691686602383
      | 254.400604378871
      | 242.676261199004
      | 229.462130210989
      | 218.075437684875
      | 207.776256300937
      | 192.222891861329
      | 178.005775209291
      | 168.578005975641
      | 157.192637101830
      | 152.195121951219]
  Saturation Dynamic1 : simulink/Discontinuities/Saturation Dynamic  OutMin=[-360]  OutMax=[360]  OutDataTypeStr=Inherit: Same as second input  OutDataType=fixdt(1, 16)  OutScaling=2^-10  DoSatur=off
  Switch : Switch  Criteria=u2 > Threshold  SaturateOnIntegerOverflow=off  InputSameDT=off
  Switch3 : Switch  SaturateOnIntegerOverflow=off  InputSameDT=off
  efficiency : Subsystem
  prod : Product
  prod1 : Product
  prod2 : Product
  rad_sec_to_rpm : Gain  Gain=60/2/pi
  tag scope: EM4FrontTorque=global, EM4Front_ElectricPower_W=global, InternalEM4FrontActivity=global
  wires:
  Switch/1 -> [InternalEM4FrontActivity]
  "1 "/1 -> Switch/1
  0/1 -> Switch/3
  EM4 Front Active/1 -> prod1/2, prod/2, Switch/2
  Memory1/1 -> Negative Motor Torque Table/1, Positive Motor Torque Table/1
  [EM4FrontTorqueCmd] -> Saturation Dynamic1/2
  efficiency/1(Electrical power [W]) -> prod1/1
  Saturation Dynamic1/1 -> prod2/1, Switch3/2, Switch3/1
  [EM4FOmega] -> rad_sec_to_rpm/1
  prod2/1 -> Switch3/3
  Positive Motor Torque Table/1 -> Saturation Dynamic1/1
  Switch3/1 -> prod/1
  Negative Motor Torque Table/1 -> Saturation Dynamic1/3
  rad_sec_to_rpm/1 -> efficiency/1(Motor speed [rpm]), Memory1/1
  prod1/1 -> [EM4Front_ElectricPower_W]
  prod/1 -> efficiency/2("Torque [Nm] "), Belt_Ratio/1
  Belt_Ratio/1 -> [EM4FrontTorque]
  [RegenFactor] -> prod2/2

== system CCModel_73/Powertrain/EM4Rear ==
  note: If Torque is positive: Motor does its best
      | If torque is negative: Case 01: SOC > 99: No Regen (Tmot = 0)
      | Case 02: SOC < 99: Regen
      | If Vehicle is stopped: No Regen Brakes
  0 : Constant
  "1 " : Constant  Value=0
  Belt_Ratio : Gain
  EM4 Rear Active : Constant  Value=EM4RearActive
  Memory1 : Memory  InheritSampleTime=on
  Negative Motor Torque Table : Lookup_n-D  NumberOfTableDimensions=1  BreakpointsForDimension1=|  Table=|  InternalRulePriority=Speed  RndMeth=Simplest
      BreakpointsForDimension1=|
      | [1
      | 300
      | 700
      | 1000
      | 1300
      | 1600
      | 1900
      | 2200
      | 2500
      | 2800
      | 3100
      | 3400
      | 3700
      | 4000
      | 4300
      | 4600
      | 4900
      | 5200
      | 5500
      | 5800
      | 6100
      | 6400
      | 6700
      | 7000
      | 7400
      | 7800
      | 8200
      | 8600
      | 8810]
      Table=|
      | [-360
      | -360
      | -360
      | -360
      | -360
      | -357.728404316261
      | -357.682405078656
      | -356.960983702214
      | -356.300227986961
      | -355.518140949330
      | -355.472141711725
      | -351.285699987009
      | -343.284814075766
      | -334.455149023278
      | -326.397812480700
      | -307.963362459085
      | -289.161940741908
      | -276.934802218937
      | -265.691686602383
      | -254.400604378871
      | -242.676261199004
      | -229.462130210989
      | -218.075437684875
      | -207.776256300937
      | -192.222891861329
      | -178.005775209291
      | -168.578005975641
      | -157.192637101830
      | -152.195121951219]
  Positive Motor Torque Table : Lookup_n-D  NumberOfTableDimensions=1  BreakpointsForDimension1=|  Table=|  InternalRulePriority=Speed  RndMeth=Simplest
      BreakpointsForDimension1=|
      | [1
      | 300
      | 700
      | 1000
      | 1300
      | 1600
      | 1900
      | 2200
      | 2500
      | 2800
      | 3100
      | 3400
      | 3700
      | 4000
      | 4300
      | 4600
      | 4900
      | 5200
      | 5500
      | 5800
      | 6100
      | 6400
      | 6700
      | 7000
      | 7400
      | 7800
      | 8200
      | 8600
      | 8810]
      Table=|
      | [360
      | 360
      | 360
      | 360
      | 360
      | 357.728404316261
      | 357.682405078656
      | 356.960983702214
      | 356.300227986961
      | 355.518140949330
      | 355.472141711725
      | 351.285699987009
      | 343.284814075766
      | 334.455149023278
      | 326.397812480700
      | 307.963362459085
      | 289.161940741908
      | 276.934802218937
      | 265.691686602383
      | 254.400604378871
      | 242.676261199004
      | 229.462130210989
      | 218.075437684875
      | 207.776256300937
      | 192.222891861329
      | 178.005775209291
      | 168.578005975641
      | 157.192637101830
      | 152.195121951219]
  Saturation Dynamic1 : simulink/Discontinuities/Saturation Dynamic  OutMin=[-360]  OutMax=[360]  OutDataTypeStr=Inherit: Same as second input  OutDataType=fixdt(1, 16)  OutScaling=2^-10  DoSatur=off
  Switch : Switch  Criteria=u2 > Threshold  SaturateOnIntegerOverflow=off  InputSameDT=off
  Switch3 : Switch  SaturateOnIntegerOverflow=off  InputSameDT=off
  efficiency : Subsystem
  prod : Product
  prod1 : Product
  prod2 : Product
  rad_sec_to_rpm : Gain  Gain=60/2/pi
  tag scope: EM4RearTorque=global, EM4rear_ElectricPower_W=global, InternalEM4RearActivity=global
  wires:
  Switch/1 -> [InternalEM4RearActivity]
  "1 "/1 -> Switch/1
  0/1 -> Switch/3
  EM4 Rear Active/1 -> Switch/2, prod1/2, prod/2
  Memory1/1 -> Negative Motor Torque Table/1, Positive Motor Torque Table/1
  [EM4RearTorqueCmd] -> Saturation Dynamic1/2
  efficiency/1(Electrical power [W]) -> prod1/1
  Saturation Dynamic1/1 -> prod2/1, Switch3/2, Switch3/1
  [EM4ROmega] -> rad_sec_to_rpm/1
  prod2/1 -> Switch3/3
  Positive Motor Torque Table/1 -> Saturation Dynamic1/1
  Switch3/1 -> prod/1
  Negative Motor Torque Table/1 -> Saturation Dynamic1/3
  rad_sec_to_rpm/1 -> efficiency/1(Motor speed [rpm]), Memory1/1
  prod1/1 -> [EM4rear_ElectricPower_W]
  prod/1 -> efficiency/2("Torque [Nm] "), Belt_Ratio/1
  Belt_Ratio/1 -> [EM4RearTorque]
  [RegenFactor] -> prod2/2
